simulink model "GFLIB_Ramp_BAM_F16"  (Simulink 8.3)
settings: Solver=ode45  StartTime=0.0  StopTime=10.0  RelTol=1e-3
undefined symbols (not defined in the file): f16RampDown, f16RampUp
settings Model: Creator=B17364  LastModifiedBy=B17364
settings OptimizationCC: ExpressionDepthLimit=2147483647
settings DebuggingCC: FcnCallInpInsideContextMsg=UseLocalSettings  StrictBusMsg=Warning

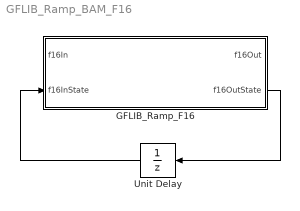
== system GFLIB_Ramp_BAM_F16 ==
  GFLIB_Ramp_F16 : Subsystem  mask(GFLIB_Ramp){f16RampUp=f16RampUp, f16RampDown=f16RampDown}
      mask help: Bit accurate model of ramp function. All parameters as well as input and output are 16bit integers.
      mask init:
      | pos = get_param(gcb, 'Position');width = pos(3) - pos(1); height = pos(4) - pos(2);tX=width/2;tY=height*0.9;
      mask Display: color('black');port_label('input',1,'f16In');port_label('input',2,'f16InState');port_label('output',1,'f16Out');port_label('output',2,'f16OutState');color('black');disp('GFLIB_Ramp_F16');color('blue');text(tX,tY, 'BAM', 'horizontalAlignment', 'center');
  Unit Delay : UnitDelay  SampleTime=-1
  wires:
  GFLIB_Ramp_F16/2(f16OutState) -> Unit Delay/1
  Unit Delay/1 -> GFLIB_Ramp_F16/2(f16InState)

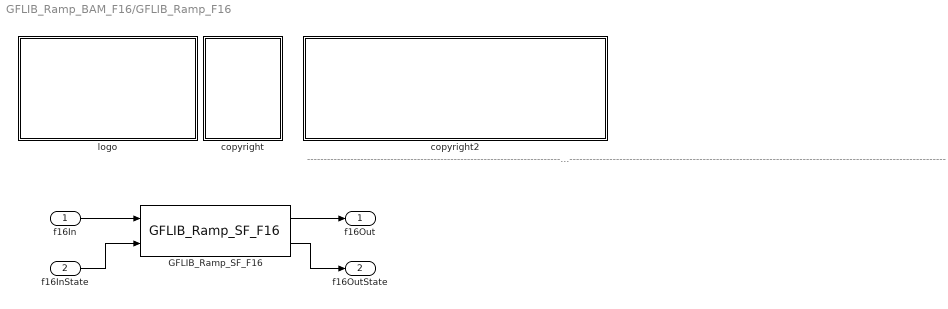
== system GFLIB_Ramp_BAM_F16/GFLIB_Ramp_F16 ==
  note: ---------------------------------------------------------------------------------------------------------------------------------------------------------------------------------------------------
  f16In : Inport
  f16InState : Inport  Port=2
  GFLIB_Ramp_SF_F16 : S-Function  FunctionName=GFLIB_Ramp_SF_F16  Parameters=f16RampUp,f16RampDown  EnableBusSupport=off
  copyright : Subsystem
      mask Display:
      | text(10,90,'FILE:');text(10,75,'DESRIPTION:')
      | text(10,60,'COPYRIGHT:')
      | text(10,45,'VERSION:')
      | text(10,30,'DATE:')
      | text(10,15,'AUTHOR:')
  copyright2 : Subsystem
      mask Display:
      | text(10,90,'GFLIB_Ramp_BAM_F16.mdl');text(10,75,'Rate of change limiter - Ramp function.');text(10,60,'Freescale')
      | text(10,45,'0.1');text(10,30,'08-Apr-2014');text(10,15,'');
  logo : Subsystem
      mask Display: image(imread('logo.jpg'))
  f16Out : Outport
  f16OutState : Outport  Port=2
  wires:
  f16In/1 -> GFLIB_Ramp_SF_F16/1
  GFLIB_Ramp_SF_F16/1 -> f16Out/1
  GFLIB_Ramp_SF_F16/2 -> f16OutState/1
  f16InState/1 -> GFLIB_Ramp_SF_F16/2

== system GFLIB_Ramp_BAM_F16/GFLIB_Ramp_F16/copyright ==

== system GFLIB_Ramp_BAM_F16/GFLIB_Ramp_F16/copyright2 ==

== system GFLIB_Ramp_BAM_F16/GFLIB_Ramp_F16/logo ==
